simulink model "default"  (R2024b)
settings: Solver=VariableStepAuto  StartTime=0.0  StopTime=10.0  RelTol=1e-3
undefined symbols (not defined in the file): Earth, Sim3dSensor, WGS84
libraries: sim3dlib x4, aerolibtransform2 x1
settings Model: Creator=ethar  LastModifiedBy=ethar

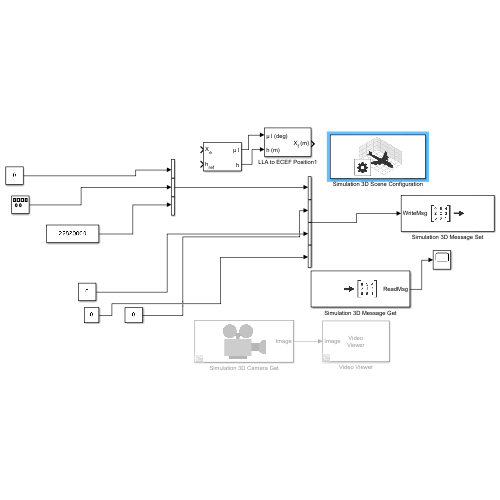
[thumbnail: Simulink's stored preview of the top-level diagram]
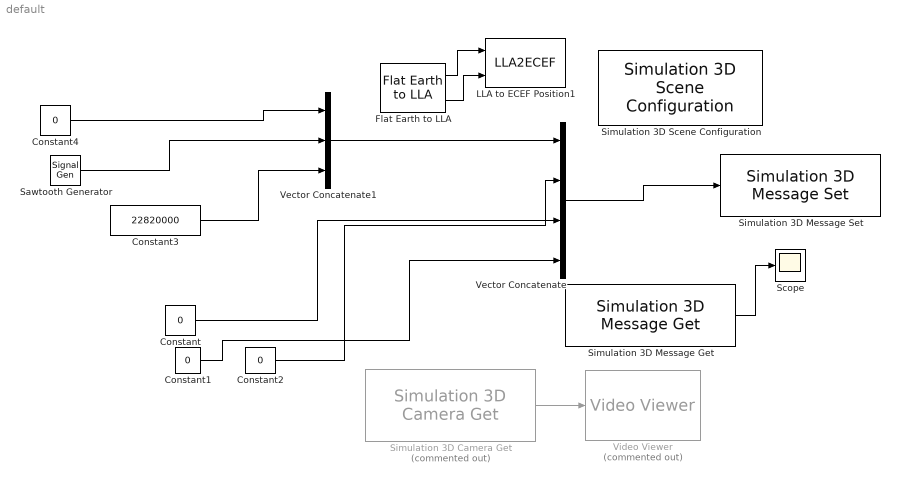
== system default ==
  Constant : Constant  Value=0
  Constant1 : Constant  Value=0  VectorParams1D=off  OutDataTypeStr=double
  Constant2 : Constant  Value=0  VectorParams1D=off  OutDataTypeStr=double
  Constant3 : Constant  Value=22820000
  Constant4 : Constant  Value=0
  Flat Earth to LLA : aerolibtransform2/Flat Earth to LLA  units=Metric (MKS)  ptype=Earth (WGS84)  F=1/298.257223563  R=6378137  refPosPort=off  LL0=[0 10]  psi=0
  LLA to ECEF Position1 : LLA2ECEF
  Sawtooth Generator : SignalGenerator  WaveForm=sawtooth  Amplitude=-360  Frequency=0.02
  Scope : Scope
  Simulation 3D Camera Get : sim3dlib/Simulation 3D Camera Get  Priority=1  Commented=on  sensorTag=Sim3dSensor�  sensorId=1  sensorName=Sim3dSensor�  vehTagList={'Scene Origin'}  vehTag=Scene Origin  mountLoc=Origin  offsetFlag=off  tmountOffset=[0, 0, 0]  rmountOffset=[0, 0, 0]  HorizontalResolution=1280  VerticalResolution=720  HorizontalFOV=60  SampleTime=-1  mountPoint=[0 0 0]  mountOrientation=[0 0 0]  aMode=0  ID=1
      settings: LibrarySourceBlock=aerolibsim3d/Simulation 3D Camera Get
  Simulation 3D Message Get : sim3dlib/Simulation 3D Message Get  Priority=1  SigName=ConeLocGet  DataType=double  MsgSize=[1, 6]  Ts=0.02  aMode=0
      settings: LibrarySourceBlock=aerolibsim3d/Simulation 3D Message Get
  Simulation 3D Message Set : sim3dlib/Simulation 3D Message Set  Priority=-1  SigName=ConeLocSet  Ts=0.02  aMode=0
      settings: LibrarySourceBlock=aerolibsim3d/Simulation 3D Message Set
  Simulation 3D Scene Configuration : sim3dlib/Simulation 3D Scene Configuration  Priority=0  ProjectFormat=Unreal Editor  SceneDesc=Airport  ProjectName=C:\Program Files\MATLAB\R2024b\toolbox\shared\sim3d_projects\automotive_project_windows\UE\WindowsNoEditor\VehicleSimulation.exe  ScenePath=/Game/Maps/HwStrght  UEProjPath=C:\Users\ethar\Simulation\Aquila\Aquila.uproject  EnableOpenDRIVE=off  vehTagList={'Custom';'Scene Origin'}  vehTag=Scene Origin  FreeCameraInitialTranslation=[-6, 0, 2]  FreeCameraDefaultInitialTranslation=[-6, 0, 2]  FreeCameraInitialRotation=[0, -15, 0]  FreeCameraDefaultInitialRotation=[0, -15, 0]  OpVisEn=off  Ts=.02  EnableWindow=on  EnableRemoteAccess=off  EnableWeather=off  SunAzimuth=90  SunAltitude=40.0  EnableGeospatialSun=off  Latitude=0  Longitude=0  Date=2023-01-01  Time=10:30:00  GeoTimeZone=-5.0  SunDaylightSaving=off  wind=1  clouds=10  EnableVolumetricClouds=off  CloudCoverage=0  CloudAltitude=6  fog=0  rain=0  RaindropsEffect=off  SnowDensity=0  EnableGeospatial=off  UseTrueOrigin=on  OriginHeight=200  OriginLatitude=0  OriginLongitude=0  MapStyle=Aerial  AdditionalAssetIDs=[]  UseAdvancedSunSky=off  SolarTime=11  TimeZone=-5  Day=21  Month=9  Year=2022  UseDaylightSavingTime=on  DSTStartDay=10  DSTStartMonth=3  DSTEndDay=3  DSTEndMonth=11  DSTSwitchHour=2  sensorTag=MainCamera1  sensorId=1  sensorName=MainCamera1  mountLoc=Origin  offsetFlag=off  tmountOffset=[0, 0, 0]  rmountOffset=[0, 0, 0]  HorizontalResolution=1280  VerticalResolution=720  HorizontalFOV=60  mountPoint=[0 0 0]  mountOrientation=[0 0 0]  aMode=0  ID=1  GeoTrigger=Inactive
      settings: LibrarySourceBlock=aerolibsim3d/Simulation 3D Scene Configuration
  Vector Concatenate : Concatenate  NumInputs=4
  Vector Concatenate1 : Concatenate  NumInputs=3
  Video Viewer : VideoViewer  Commented=on  FigPos=[1 814 1536 716]
  wires:
  Vector Concatenate/1 -> Simulation 3D Message Set/1
  Simulation 3D Message Get/1 -> Scope/1
  Simulation 3D Camera Get/1 -> Video Viewer/1
  Constant1/1 -> Vector Concatenate/4
  Constant2/1 -> Vector Concatenate/2
  Constant3/1 -> Vector Concatenate1/3
  Flat Earth to LLA/1 -> LLA to ECEF Position1/1
  Flat Earth to LLA/2 -> LLA to ECEF Position1/2
  Vector Concatenate1/1 -> Vector Concatenate/1
  Constant/1 -> Vector Concatenate/3
  Sawtooth Generator/1 -> Vector Concatenate1/2
  Constant4/1 -> Vector Concatenate1/1
